simulink model "model_1"  (R2014a)
settings: Solver=ode3  StartTime=0.0  StopTime=3000  FixedStep=0.1  RelTol=1e-3
settings Model: Creator=Павел  LastModifiedBy=Павел
settings DataIOCC: InspectSignalLogs=on

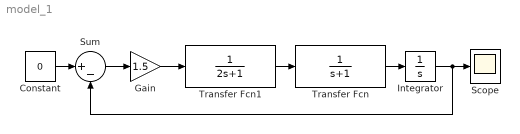
== system model_1 ==
  Constant : Constant  Value=0
  Gain : Gain  Gain=1.5
  Integrator : Integrator  InitialCondition=1
  Scope : Scope
      settings: TimeRange=30
  Sum : Sum  Inputs=|+-
  Transfer Fcn : TransferFcn  Denominator=[1 1]
  Transfer Fcn1 : TransferFcn  Denominator=[2 1]
  wires:
  Sum/1 -> Gain/1
  Constant/1 -> Sum/1
  Gain/1 -> Transfer Fcn1/1
  Transfer Fcn1/1 -> Transfer Fcn/1
  Transfer Fcn/1 -> Integrator/1
  Integrator/1 -> Sum/2, Scope/1
